simulink library "Collector_Unglazed_CONF"  (R2016b)
settings: Solver=ode45  StartTime=0.0  StopTime=10.0  RelTol=1e-3  EnableMultiTasking=on
undefined symbols (not defined in the file): Acol, path_carnot, Qdot, THBin, THBout
libraries: carnot x2
settings Model: Creator=lena.frank  LastModifiedBy=drhf
settings DataIOCC: LimitDataPoints=on  SaveFormat=Array  SignalLoggingSaveFormat=ModelDataLogs
settings OptimizationCC: ExpressionDepthLimit=2147483647  LifeSpan=inf
settings DebuggingCC: UnderspecifiedInitializationDetection=Classic  MergeDetectMultiDrivingBlocksExec=none  SolverPrmCheckMsg=warning  FcnCallInpInsideContextMsg=warning  StateNameClashWarn=warning  SFUnexpectedBacktrackingDiag=warning  SFNoUnconditionalDefaultTransitionDiag=warning  SFExecutionAtInitializationDiag=none
settings HardwareCC: ProdBitPerPointer=32  ProdBitPerSizeT=32  ProdBitPerPtrDiffT=32  ProdLargestAtomicFloat=None  ProdIntDivRoundTo=Undefined  ProdEndianess=Unspecified  ProdWordSize=32  ProdHWDeviceType=32-bit Generic
settings ModelReferenceCC: PropagateSignalLabelsOutOfModel=off
settings GRTTargetCC: TargetLangStandard=C89/C90 (ANSI)  GeneratePreprocessorConditionals=Disable all  CombineOutputUpdateFcns=off  GRTInterface=on
settings ConfigComp: CovMetricSettings=dw  CovHtmlReporting=on  CovSaveCumulativeToWorkspaceVar=on  CovSaveSingleToWorkspaceVar=on  CovExternalEMLEnable=off

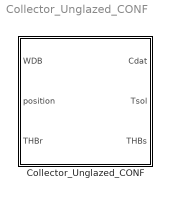
== system Collector_Unglazed_CONF ==
  Collector_Unglazed_CONF : Subsystem  mask(Unglazed solar thermal collector (CONFIGURATED)){tini=20, Ncollector=1, PathName=fullfile(path_carnot('libsl'),'Source','Solar_Thermal','Collector_Unglazed_CONF','parameter_set'), FileName='DefaultCollectorUnglazed.mat', userPath=off, userParam=off, acol=2.5, len=2.3, nodes=5, fta=0.75, eps=0.9, u0l=4, u0c=10, u0g=4, u1l=3, u1c=3, u1g=1.5, u1e=0.01, hi=100, capa=7000, capf=2000, SensorTimeConstant=10, dplin=10, dpqua=10}
      mask prompts: tini "Initial temperature [°C]"; Ncollector "Number of collectors in parallel"; PathName "Path"; FileName "Parameter set"; userPath "Edit path and name of parameter set"; userParam "User defined parameters"; acol "Collector surface (aperture) in [m²]"; len "Length between inlet and outlet [m]"; nodes "Number of nodes (>=2)"; fta "Absorption coefficient of the absorber [-]"; eps "Thermal emissivity of the absorber (0..1)"; u0l "U0L heat transfer for losses [W/(m²*K)]"; u0c "U0C heat transfer for condensation [W/(m²*K)]"; u0g "U0G heat transfer for gains [W/(m²*K)]"; u1l "U1L wind dependent heat transfer for losses [W/(m²*K*m/s)]"; u1c "U1C wind dependent heat transfer for condensation [W/(m²*K*m/s)]"; u1g "U1G wind dependent heat transfer for gains [W/(m²*K*m/s)]"; u1e "U1E wind dependancy of optical efficiency in W/(m²*m/s)"; hi "HI heat transfer between collector and tube [W/(m²*K)]"; capa "Effective heat capacity of absorber [J/(m²*K)]"; capf "Effective heat capacity of fluid [J/(m²*K)]"; SensorTimeConstant "Time constant of temperature sensor [s]"; dplin "Linear pressure drop in Pa/(kg/s)"; dpqua "Quadratic pressure drop in Pa/(kg/s)²"
      mask help:
      | N-node model, parameters according to EN 12975.
      | Use of buttons in the "Picking a file" frame:
      | 1) "Carnot public data" choses a parameter file from the public data folder in Carnot. The "Path" is set to the public data folder.
      | 2) "Carnot internal data" choses a parameter file from the internal data folder in Carnot. The "Path" is set to the internal data folder.
      | 3) "From selected path" choses a parameter file from the "Path".
      | Allow editing "File" and "Path" with the checkbox. Be aware that the buttons in the "Picking a file" frame will anyway overwrite the edited values.
      mask init:
      | [ok, param] = CarnotCallbacks_CollectorUnglazedConf('SetParameters',gcbh,PathName,FileName);
      mask Help: web(fullfile(path_carnot('help'),'Collector_Unglazed.html'),'-helpbrowser')
      mask TypeOptions tini: Collector_Unglazed/tini | T_Sensor1/t0
      mask TypeOptions Ncollector: Ncollector/Value | Gain/Gain | Gain3/Gain
      mask Callback userPath: [ok, param] = CarnotCallbacks_CollectorUnglazedConf('UserEdit',gcbh);
      mask Callback userParam: [ok, param] = CarnotCallbacks_CollectorUnglazedConf('UserEdit',gcbh);
      mask TypeOptions acol: Collector_Unglazed/acol
      mask TypeOptions len: Collector_Unglazed/len
      mask TypeOptions nodes: Collector_Unglazed/nodes
      mask TypeOptions fta: Collector_Unglazed/fta
      mask TypeOptions eps: Collector_Unglazed/e_sky
      mask TypeOptions u0l: Collector_Unglazed/uc0loss
      mask TypeOptions u0c: Collector_Unglazed/uc0
      mask TypeOptions u0g: Collector_Unglazed/uc0gain
      mask TypeOptions u1l: Collector_Unglazed/uc1loss
      mask TypeOptions u1c: Collector_Unglazed/uc1
      mask TypeOptions u1g: Collector_Unglazed/uc1gain
      mask TypeOptions u1e: Collector_Unglazed/uc1eta0
      mask TypeOptions hi: Collector_Unglazed/hi
      mask TypeOptions capa: Collector_Unglazed/c_abs
      mask TypeOptions capf: Collector_Unglazed/c_fl
      mask TypeOptions SensorTimeConstant: T_Sensor1/tc
      mask TypeOptions dplin: Collector_Unglazed/lin
      mask TypeOptions dpqua: Collector_Unglazed/qua
      mask DialogControl Control3 Prompt: Carnot public data
      mask DialogControl Control3 Callback: [ok, file] = CarnotCallbacks_CollectorUnglazedConf('GetFilename',gcbh, 'public');
      mask DialogControl Control4 Prompt: Carnot internal data
      mask DialogControl Control4 Callback: [ok, file] = CarnotCallbacks_CollectorUnglazedConf('GetFilename',gcbh, 'internal');
      mask DialogControl Control2 Prompt: Selected path
      mask DialogControl Control2 Callback: [ok, file] = CarnotCallbacks_CollectorUnglazedConf('GetFilename',gcbh, 'selected');
      mask DialogControl Control6 Prompt: Save in Carnot internal data
      mask DialogControl Control6 Callback: [ok, param] = CarnotCallbacks_CollectorUnglazedConf('SaveFilename',gcbh, 'internal','USTC');
      mask DialogControl Control5 Prompt: Save in selected path
      mask DialogControl Control5 Callback: [ok, param] = CarnotCallbacks_CollectorUnglazedConf('SaveFilename',gcbh, 'selected','USTC');
      mask Display:
      | % user defined picture file
      | picfile = fullfile(path_carnot('intlibsl'), ...
      |     'Source','Solar_Thermal','Collector_Unglazed_CONF','parameter_set', ...
      |      'Collector_CONF.jpg');
      | 
      | pic = false;
      | 
      | % show internal picture if defined
      | if ~BlockIsInCarnotLibrary    % if not located in library any more
      |     if exist(picfile)
      |         image(imread(picfile), [0.1, 0, 0.9, 1])
      |         set_param(gcb, 'BackgroundColor', 'White')
      |         pic = true;
      |     end
      | end
      | 
      | if ~pic % show public picture
      |     plot([0,70,70,0,0]/100,[-0,-0,5,5,-0]/100,[30,30,100,100,30]/100,...
      |         [100,94,94,100,100]/100,[32,1]/100,[94,5]/100,[40,10]/100,...
      |         [94,5]/100,[49,19]/100,[94,5]/100,[57,27]/100,[94,5]/100,[65,35]/100,...
      |         [94,5]/100,[73,43]/100,[94,5]/100,[82,51]/100,[94,5]/100,[90,60]/100,...
      |         [94,5]/100,[98,68]/100,[94,5]/100)
      |     set_param(gcb, 'BackgroundColor', 'Yellow')
      | end
      | 
      | % Show port labels: same as port labels in the subsystem,
      | % but display with a picture covers the text. Have to reprint it.
      | % port_label('input',1,'WDB')
      | % port_label('input',2,'position')
      | % port_label('input',3,'THBr')
      | % port_label('output',1,'Cdat')
      | % port_label('output',2,'Tsol')
      | % port_label('output',3,'THBs')

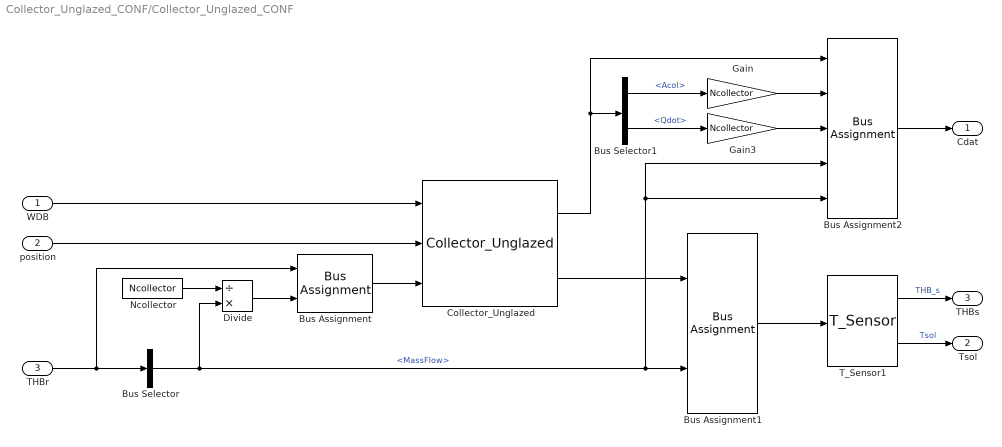
== system Collector_Unglazed_CONF/Collector_Unglazed_CONF ==
  WDB : Inport
  position : Inport  Port=2
  THBr : Inport  Port=3
  Bus Assignment : BusAssignment  AssignedSignals=MassFlow
  Bus Assignment1 : BusAssignment  AssignedSignals=MassFlow
  Bus Assignment2 : BusAssignment  AssignedSignals=Acol,Qdot,THBin.MassFlow,THBout.MassFlow
  Bus Selector : BusSelector  OutputSignals=MassFlow
  Bus Selector1 : BusSelector  OutputSignals=Acol,Qdot
  Collector_Unglazed : carnot/Source/Solar_Thermal/Collector_Unglazed  acol=acol  len=len  fta=fta  e_sky=eps  uc0=u0c  uc1=u1c  uc0loss=u0l  uc1loss=u1l  uc0gain=u0g  uc1gain=u1g  uc1eta0=u1e  hi=hi  c_abs=capa  c_fl=capf  lin=dplin  qua=dpqua  tini=tini  nodes=nodes
  Divide : Product  Inputs=/*
  Gain : Gain  Gain=Ncollector
  Gain3 : Gain  Gain=Ncollector
  Ncollector : Constant  Value=Ncollector
  T_Sensor1 : carnot/Control/T_Sensor  tc=SensorTimeConstant  t0=tini
  Cdat : Outport
  Tsol : Outport  Port=2
  THBs : Outport  Port=3
  wires:
  T_Sensor1/2 -> Tsol/1  "Tsol"
  T_Sensor1/1 -> THBs/1  "THB_s"
  Collector_Unglazed/2 -> Bus Assignment1/1
  WDB/1 -> Collector_Unglazed/1
  position/1 -> Collector_Unglazed/2
  THBr/1 -> Bus Assignment/1, Bus Selector/1
  Collector_Unglazed/1 -> Bus Assignment2/1, Bus Selector1/1
  Bus Assignment/1 -> Collector_Unglazed/3
  Bus Assignment1/1 -> T_Sensor1/1
  Bus Selector/1 -> Divide/2, Bus Assignment2/5, Bus Assignment2/4, Bus Assignment1/2  "<MassFlow>"
  Ncollector/1 -> Divide/1
  Divide/1 -> Bus Assignment/2
  Bus Selector1/1 -> Gain/1  "<Acol>"
  Bus Selector1/2 -> Gain3/1  "<Qdot>"
  Gain/1 -> Bus Assignment2/2
  Gain3/1 -> Bus Assignment2/3
  Bus Assignment2/1 -> Cdat/1
